simulink model "BobsatElectricalV1"  (R2025b)
settings: Solver=VariableStepAuto  StartTime=0.0  StopTime=10.0  RelTol=1e-3
undefined symbols (not defined in the file): BatterySupportPower_W, BuckConverter_Efficiency, LoadPower_ADCS_W, LoadPower_COMM_W, LoadPower_DBC_W, LoadPower_Payload_W, MPPT_Controller_Efficiency, Payload_DutyCycle_Fraction, SolarArray_TotalPower_W
settings Model: Creator=synci  LastModifiedBy=synci

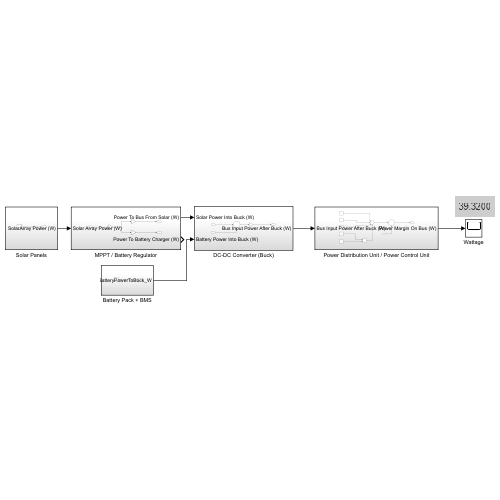
[thumbnail: Simulink's stored preview of the top-level diagram]
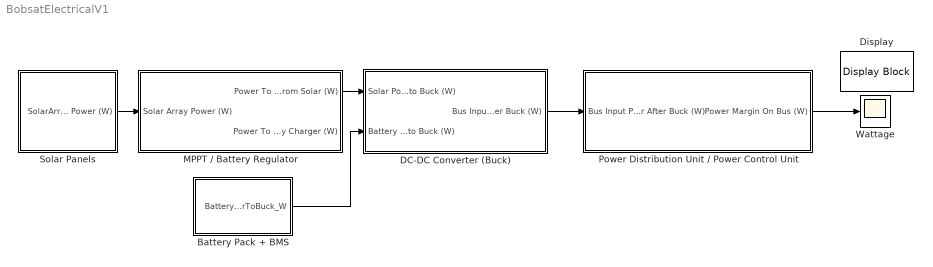
== system BobsatElectricalV1 ==
  Battery Pack + BMS : Subsystem
  DC-DC Converter (Buck) : Subsystem
  Display : DisplayBlock  LabelPosition=Hide  Transparency=1  GridColor=[0.502, 0.502, 0.502]
  MPPT / Battery Regulator : Subsystem
  Power Distribution Unit / Power Control Unit : Subsystem
  Solar Panels : Subsystem
  Wattage : Scope
      settings: ActiveDisplayYMinimum=-1  ActiveDisplayYMaximum=1
  wires:
  DC-DC Converter (Buck)/1(Bus Input Power After Buck (W)) -> Power Distribution Unit / Power Control Unit/1(Bus Input Power After Buck (W))
  MPPT / Battery Regulator/1(Power To Bus From Solar (W)) -> DC-DC Converter (Buck)/1(Solar Power Into Buck (W))
  Battery Pack + BMS/1(BatteryPowerToBuck_W) -> DC-DC Converter (Buck)/2(Battery Power Into Buck (W))
  Power Distribution Unit / Power Control Unit/1(Power Margin On Bus (W)) -> Wattage/1
  Solar Panels/1(SolarArray Power (W)) -> MPPT / Battery Regulator/1(Solar Array Power (W))

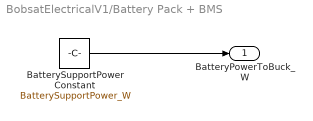
== system BobsatElectricalV1/Battery Pack + BMS ==
  BatterySupportPowerConstant : Constant  Value=BatterySupportPower_W
  BatteryPowerToBuck_W : Outport
  wires:
  BatterySupportPowerConstant/1 -> BatteryPowerToBuck_W/1

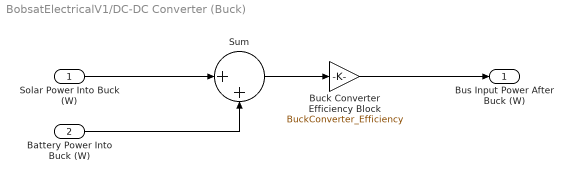
== system BobsatElectricalV1/DC-DC Converter (Buck) ==
  Solar Power Into Buck (W) : Inport
  Battery Power Into Buck (W) : Inport  Port=2
  Buck Converter Efficiency Block : Gain  Gain=BuckConverter_Efficiency
  Sum : Sum  Inputs=|++
  Bus Input Power After Buck (W) : Outport
  wires:
  Solar Power Into Buck (W)/1 -> Sum/1
  Battery Power Into Buck (W)/1 -> Sum/2
  Sum/1 -> Buck Converter Efficiency Block/1
  Buck Converter Efficiency Block/1 -> Bus Input Power After Buck (W)/1

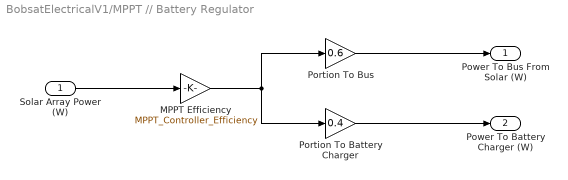
== system BobsatElectricalV1/MPPT // Battery Regulator ==
  Solar Array Power (W) : Inport
  MPPT Efficiency : Gain  Gain=MPPT_Controller_Efficiency
  Portion To Battery Charger : Gain  Gain=0.4
  Portion To Bus : Gain  Gain=0.6
  Power To Bus From Solar (W) : Outport
  Power To Battery Charger (W) : Outport  Port=2
  wires:
  Solar Array Power (W)/1 -> MPPT Efficiency/1
  MPPT Efficiency/1 -> Portion To Battery Charger/1, Portion To Bus/1
  Portion To Bus/1 -> Power To Bus From Solar (W)/1
  Portion To Battery Charger/1 -> Power To Battery Charger (W)/1

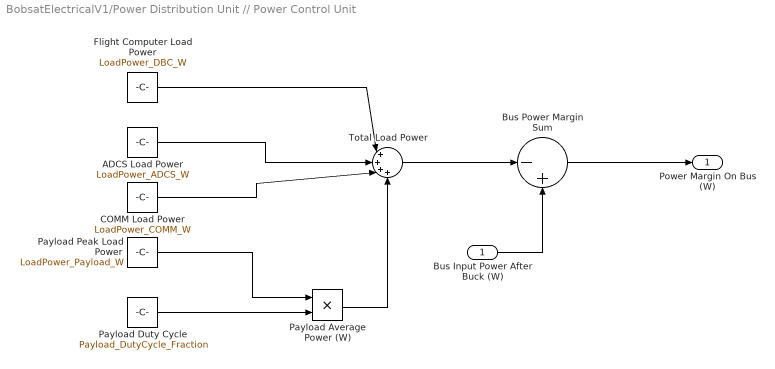
== system BobsatElectricalV1/Power Distribution Unit // Power Control Unit ==
  Bus Input Power After Buck (W) : Inport
  ADCS Load Power : Constant  Value=LoadPower_ADCS_W
  Bus Power Margin Sum : Sum  Inputs=|-+
  COMM Load Power : Constant  Value=LoadPower_COMM_W
  Flight Computer Load Power : Constant  Value=LoadPower_DBC_W
  Payload Average Power (W) : Product
  Payload Duty Cycle : Constant  Value=Payload_DutyCycle_Fraction
  Payload Peak Load Power : Constant  Value=LoadPower_Payload_W
  Total Load Power : Sum  Inputs=|++++
  Power Margin On Bus (W) : Outport
  wires:
  Payload Duty Cycle/1 -> Payload Average Power (W)/2
  Payload Peak Load Power/1 -> Payload Average Power (W)/1
  Flight Computer Load Power/1 -> Total Load Power/1
  ADCS Load Power/1 -> Total Load Power/2
  COMM Load Power/1 -> Total Load Power/3
  Payload Average Power (W)/1 -> Total Load Power/4
  Total Load Power/1 -> Bus Power Margin Sum/1
  Bus Input Power After Buck (W)/1 -> Bus Power Margin Sum/2
  Bus Power Margin Sum/1 -> Power Margin On Bus (W)/1

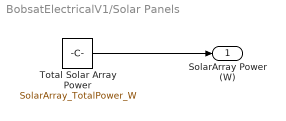
== system BobsatElectricalV1/Solar Panels ==
  Total Solar Array Power : Constant  Value=SolarArray_TotalPower_W
  SolarArray Power (W) : Outport
  wires:
  Total Solar Array Power/1 -> SolarArray Power (W)/1
